simulink model "AMR_MotorControlUnit_23b"  (R2024a)
settings: Solver=FixedStepAuto  StartTime=0.0  StopTime=inf  FixedStep=1e-3  RelTol=1e-3
model workspace (MAT data in the model file):
  RTK_health_condition = 30
  min_motor_rpm = 30
settings Model: DataDictionary=configuration_dictionary.sldd  Creator=matlab.cut  LastModifiedBy=matlab.cut
settings SolverCC: ConcurrentTasks=on  PositivePriorityOrder=on
settings OptimizationCC: BlockReduction=off  DefaultParameterBehavior=Inlined  OptimizeBlockIOStorage=off
settings DebuggingCC: TasksWithSamePriorityMsg=none
settings HardwareCC: ProdBitPerLong=64  ProdLongLongMode=on  ProdHWDeviceType=Intel->x86-64 (Linux 64)
settings ModelReferenceCC: ModelReferenceNumInstancesAllowed=Single
settings SFSimCC: MATLABDynamicMemAlloc=off
settings RTWCC: Description=Speedgoat Real-Time Target Machine  SystemTargetFile=speedgoat.tlc  TemplateMakefile=slrealtime_default_tmf  Toolchain=Simulink Real-Time Toolchain  BuildConfiguration=Faster Runs  CodeExecutionProfiling=on  TargetLang=C++  GPUComputeCapability=3.5
settings CodeAppCC: MaxIdLength=127
settings SimulinkRealTimeTargetCC: InstructionSetFMA=off  LogToMDFFile=off

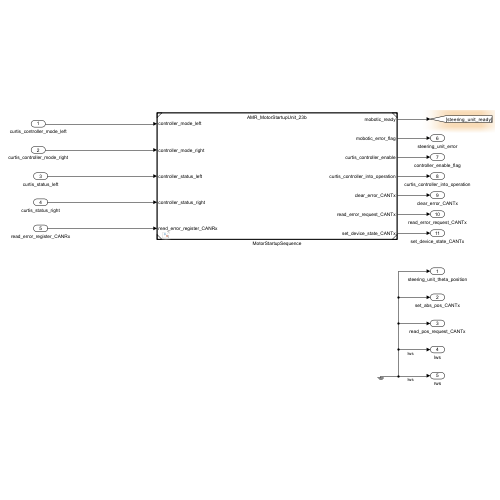
[thumbnail: Simulink's stored preview of the top-level diagram]
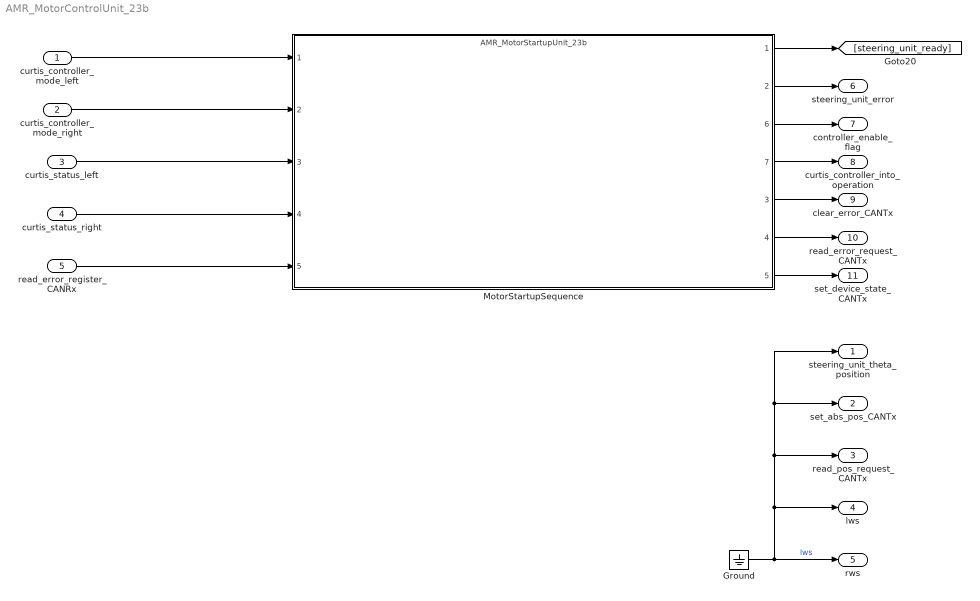
== system AMR_MotorControlUnit_23b ==
  curtis_controller_mode_left : Inport
  curtis_controller_mode_right : Inport  Port=2
  curtis_status_left : Inport  Port=3
  curtis_status_right : Inport  Port=4
  read_error_register_CANRx : Inport  Port=5
  Ground : Ground
  MotorStartupSequence : ModelReference  ModelNameDialog=AMR_MotorStartupUnit_23b.slx  SimulationMode=Normal  ModelReferenceVersion=2.15
      settings: PortSchema="{\"entries\":[{\"content\":{\"sides\":[{\"content\":{\"connectorIds\":[\"In1\",\"In2\",\"In3\",\"In4\",\"In5\"]},\"type\":\"ConnectorPlacement.EquallySpacedRectSide\",\"uuid\":\"60542e90-c7e2-44d4-b42e-e1f7bbf2f5e1\"},{\"content\":{\"connectorIds\":[\"Out1\",\"Out2\",\"Out6\",\"Out7\",\"Out3\",\"Out4\",\"Out5\"],\"side\":\"RIGHT\"},\"type\":\"ConnectorPlacement.EquallySpacedRectSide\",\"uuid\":\"46c4052c-7563-41d8-bb6f-81b3d3992952\"},{\"content\":{\"side\":\"TOP\"},\"type\":\"ConnectorPlacement.EquallySpacedRectSide\",\"uuid\":\"c8f4b4e7-61ba-46f6-bc89-74f082c59f99\"}]},\"type\":\"ConnectorPlacement.EquallySpacedConnector\",\"uuid\":\"c4be2919-7166-47d8-b000-027784c45f40\"}],\"packageUris\":[\"http://schema.mathworks.com/mf0/Connector/R2020b\"],\"version\":\"1.0\"}"
  steering_unit_theta_position : Outport
  set_abs_pos_CANTx : Outport  Port=2
  read_pos_request_CANTx : Outport  Port=3
  lws : Outport  Port=4
  rws : Outport  Port=5
  steering_unit_error : Outport  Port=6
  controller_enable_flag : Outport  Port=7
  curtis_controller_into_operation : Outport  Port=8
  clear_error_CANTx : Outport  Port=9
  read_error_request_CANTx : Outport  Port=10
  set_device_state_CANTx : Outport  Port=11
  wires:
  curtis_status_right/1 -> MotorStartupSequence/4
  MotorStartupSequence/1 -> [steering_unit_ready]
  curtis_controller_mode_right/1 -> MotorStartupSequence/2
  curtis_controller_mode_left/1 -> MotorStartupSequence/1
  Ground/1 -> steering_unit_theta_position/1, set_abs_pos_CANTx/1, read_pos_request_CANTx/1, lws/1, rws/1  "lws"
  curtis_status_left/1 -> MotorStartupSequence/3
  MotorStartupSequence/2 -> steering_unit_error/1
  read_error_register_CANRx/1 -> MotorStartupSequence/5
  MotorStartupSequence/3 -> clear_error_CANTx/1
  MotorStartupSequence/4 -> read_error_request_CANTx/1
  MotorStartupSequence/5 -> set_device_state_CANTx/1
  MotorStartupSequence/6 -> controller_enable_flag/1
  MotorStartupSequence/7 -> curtis_controller_into_operation/1
